simulink model "bb2"  (R2016b)
settings: Solver=VariableStepAuto  StartTime=0.0  StopTime=10.0  RelTol=1e-3
settings Model: Creator=ayase-252  LastModifiedBy=ayase-252

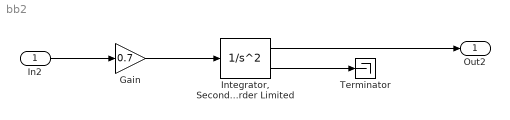
== system bb2 ==
  In2 : Inport
  Gain : Gain  Gain=0.7
  "Integrator, Second-Order Limited" : SecondOrderIntegrator  LimitX=on  UpperLimitX=0.4  LowerLimitX=0  LimitDXDT=on
  Terminator : Terminator
  Out2 : Outport
  wires:
  In2/1 -> Gain/1
  "Integrator, Second-Order Limited"/1 -> Out2/1
  Gain/1 -> "Integrator, Second-Order Limited"/1
  "Integrator, Second-Order Limited"/2 -> Terminator/1
